simulink model "clock_recovery_3"  (Simulink 7.4)
settings: Solver=ode45  StartTime=0.0  StopTime=1e-5  MaxStep=.1/bit_rate  RelTol=1e-3
PreLoadFcn:
  | bit_rate=9.953e9;   % bits per second
libraries: simulink x7, dspsigops x6, dspsigattribs x4, commblksprivate x2, dspstat3 x2, commrandsrc2 x1, dspbuff3 x1, dspsnks4 x1
settings Model: Creator=dbenson  LastModifiedBy=Dick
settings SolverCC: ZeroCrossControl=EnableAll
settings OptimizationCC: InitFltsAndDblsToZero=on

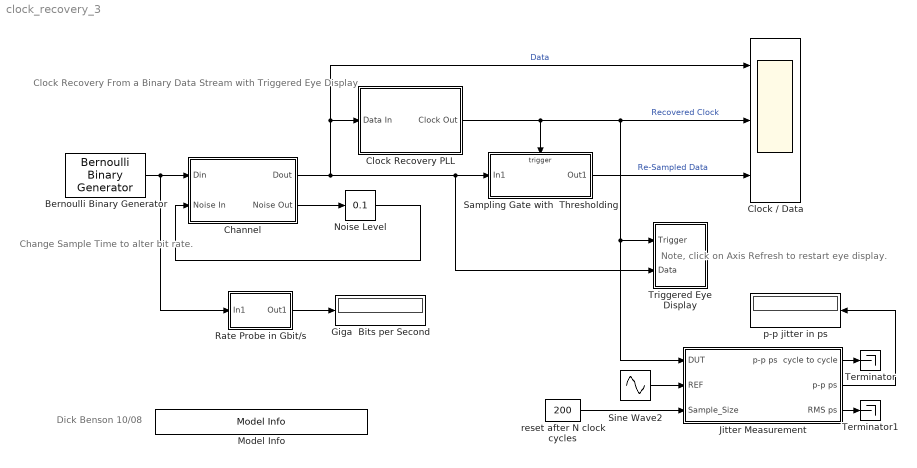
== system clock_recovery_3 ==
  note: Clock Recovery From a Binary Data Stream
      | with
      | Triggered Eye Display
  note: Note, click on Axis Refresh
      | to restart eye display.
  note: Dick Benson
      | 10/08
  note: Change Sample Time
      | to alter bit rate.
  Bernoulli Binary Generator : commrandsrc2/Bernoulli Binary Generator  DialogController=commDDGCreate  DialogControllerArgs=DataTag0  SystemSampleTime=-1  P=0.5  seed=21  Ts=1.001/ bit_rate  frameBased=off  sampPerFrame=1  orient=off  outDataType=boolean
  Channel : Subsystem
  "Clock / Data " : Scope  NumInputPorts=3
      settings: TimeRange=2.009444388626545e-010  YMin=-1~-0.2~-0.2  YMax=1~1.2~1.2
  Clock Recovery PLL : Subsystem
  Giga  Bits per Second : Display
  "Jitter Measurement " : Subsystem
  Model Info : simulink/Model-Wide Utilities/Model Info  SystemSampleTime=-1  InitialBlockCM=None  BlockCM=None  Frame=on  DisplayStringWithTags=Copywrite 2008-2010 The MathWorks, Inc.  HorizontalTextAlignment=Center  LeftAlignmentValue=0.5  SourceBlockDiagram=clock_recovery_3  TagMaxNumber=20
  Noise Level : simulink/Math Operations/Slider Gain  SystemSampleTime=-1  low=0  gain=0.1  high=1
  Rate Probe in Gbit/s : Subsystem
  Sampling Gate with  Thresholding : Subsystem
  Sine Wave2 : Sin  Amplitude=1  Bias=0  Frequency=2*pi*bit_rate  Phase=0  Samples=10  SampleTime=0  Offset=0
  Terminator : Terminator
  Terminator1 : Terminator
  Triggered Eye Display : Subsystem
  p-p jitter in ps : Display
  reset after N clock cycles : Constant  Value=200  VectorParams1D=off  OutDataType=sfix(16)  OutScaling=2^0
  wires:
  Clock Recovery PLL/1(Clock Out) -> Sampling Gate with  Thresholding/Trigger, "Clock / Data "/2, Triggered Eye Display/1(Trigger), "Jitter Measurement "/1(DUT)  "Recovered Clock"
  Bernoulli Binary Generator/1 -> Channel/1(Din), Rate Probe in Gbit/s/1(In1)
  Channel/1(Dout) -> Clock Recovery PLL/1(Data In), "Clock / Data "/1, Sampling Gate with  Thresholding/1(In1), Triggered Eye Display/2(Data)  "Data"
  Sampling Gate with  Thresholding/1(Out1) -> "Clock / Data "/3  "Re-Sampled Data"
  Rate Probe in Gbit/s/1(Out1) -> Giga  Bits per Second/1
  Sine Wave2/1 -> "Jitter Measurement "/2(REF)
  "Jitter Measurement "/2(p-p ps) -> p-p jitter in ps/1
  reset after N clock cycles/1 -> "Jitter Measurement "/3(Sample_Size)
  Channel/2(Noise Out) -> Noise Level/1
  Noise Level/1 -> Channel/2(Noise In)
  "Jitter Measurement "/1(p-p ps  cycle to cycle) -> Terminator/1
  "Jitter Measurement "/3(RMS ps) -> Terminator1/1

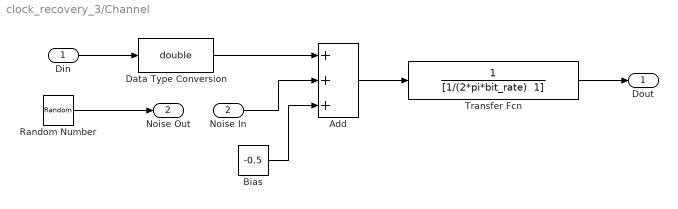
== system clock_recovery_3/Channel ==
  Din : Inport
  Noise In : Inport  Port=2
  Add : Sum  Inputs=+++  OutDataType=sfix(16)  OutScaling=2^-10
  Bias : Constant  Value=-0.5  OutDataType=sfix(16)  OutScaling=2^0
  Data Type Conversion : DataTypeConversion  OutDataTypeMode=double  OutDataType=sfix(16)  OutScaling=2^0  OutDataTypeStr=double
  Random Number : RandomNumber  SampleTime=0
  Transfer Fcn : TransferFcn  Denominator="[1/(2*pi*bit_rate)  1]"
  Dout : Outport
  Noise Out : Outport  Port=2
  wires:
  Din/1 -> Data Type Conversion/1
  Add/1 -> Transfer Fcn/1
  Data Type Conversion/1 -> Add/1
  Transfer Fcn/1 -> Dout/1
  Random Number/1 -> Noise Out/1
  Noise In/1 -> Add/2
  Bias/1 -> Add/3

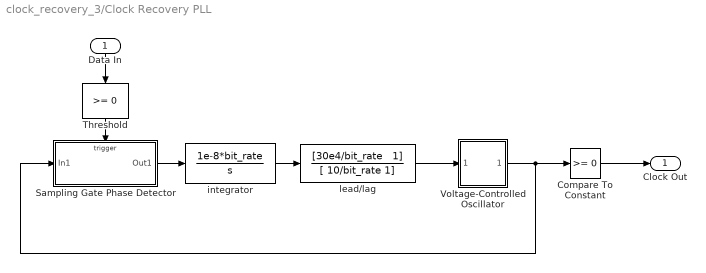
== system clock_recovery_3/Clock Recovery PLL ==
  Data In : Inport
  Compare To Constant : simulink/Logic and Bit Operations/Compare To Constant  SystemSampleTime=-1  relop=>=  const=0  LogicOutDataTypeMode=boolean  ZeroCross=off
  Sampling Gate Phase Detector : Subsystem
  Threshold : simulink/Logic and Bit Operations/Compare To Constant  SystemSampleTime=-1  relop=>=  const=0  LogicOutDataTypeMode=boolean  ZeroCross=off
  Voltage-Controlled Oscillator : Subsystem  mask(Voltage-Controlled Oscillator){Ac=1, Fc=bit_rate, Kc=bit_rate, Ph=0}
      mask prompts: Ac "Output amplitude:"; Fc "Oscillation frequency (Hz):"; Kc "Input sensitivity:"; Ph "Initial phase (rad):"
      mask help: Generate a continuous-time output signal whose frequency changes in response to the amplitude variations of the input signal. The input signal must be a sample-based scalar.
      mask init:
      | if ((length(Ac)~=1) | (length(Fc)~=1) | (length(Ph)~=1) | (length(Kc)~=1) )error('Mask parameters must be scalar values.');end;
      | pi2=2*pi;
      mask Help: helpview(commbhelp)
      mask Display: disp('VCO')
  integrator : TransferFcn  Numerator=1e-8*bit_rate  Denominator=[1 0]
  lead/lag : TransferFcn  Numerator="[30e4/bit_rate   1]"  Denominator=[ 10/bit_rate 1]
  Clock Out : Outport
  wires:
  lead/lag/1 -> Voltage-Controlled Oscillator/1(in_1)
  Voltage-Controlled Oscillator/1(out_1) -> Sampling Gate Phase Detector/1(In1), Compare To Constant/1
  integrator/1 -> lead/lag/1
  Sampling Gate Phase Detector/1(Out1) -> integrator/1
  Threshold/1 -> Sampling Gate Phase Detector/Trigger
  Data In/1 -> Threshold/1
  Compare To Constant/1 -> Clock Out/1

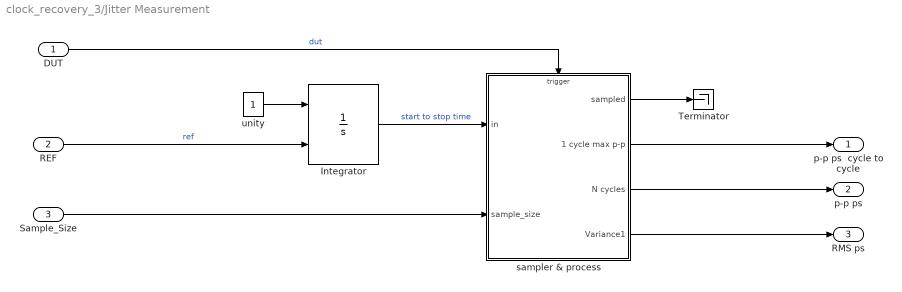
== system clock_recovery_3/Jitter Measurement  ==
  DUT : Inport  OutDataType=sfix(16)  OutScaling=2^0
  REF : Inport  Port=2  OutDataType=sfix(16)  OutScaling=2^0
  Sample_Size : Inport  Port=3  OutDataType=sfix(16)  OutScaling=2^0
  Integrator : Integrator  ExternalReset=rising
  Terminator : Terminator
  sampler & process : Subsystem  TreatAsAtomicUnit=on
  unity : Constant  OutDataTypeMode=double  OutDataType=sfix(16)  OutScaling=2^0  OutDataTypeStr=double
  p-p ps  cycle to cycle : Outport  OutDataType=sfix(16)  OutScaling=2^0
  p-p ps : Outport  Port=2  OutDataType=sfix(16)  OutScaling=2^0
  RMS ps : Outport  Port=3  OutDataType=sfix(16)  OutScaling=2^0
  wires:
  DUT/1 -> sampler & process/Trigger  "dut"
  REF/1 -> Integrator/2  "ref"
  Integrator/1 -> sampler & process/1(in)  "start to stop time"
  Sample_Size/1 -> sampler & process/2(sample_size)
  sampler & process/3(N cycles) -> p-p ps/1
  sampler & process/4(Variance1) -> RMS ps/1
  unity/1 -> Integrator/1
  sampler & process/2(1 cycle max p-p) -> p-p ps  cycle to cycle/1
  sampler & process/1(sampled) -> Terminator/1

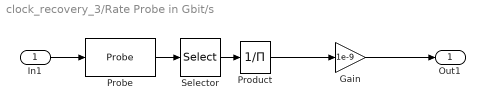
== system clock_recovery_3/Rate Probe in Gbit/s ==
  In1 : Inport
  Gain : Gain  Gain=1e-9  ParameterDataType=sfix(16)  ParameterScaling=2^0  OutDataType=sfix(16)  OutScaling=2^0
  Probe : Probe  ProbeWidth=off  ProbeComplexSignal=off
  Product : Product  Inputs=/  OutDataType=sfix(16)  OutScaling=2^0  RndMeth=Zero
  Selector : Selector  InputPortWidth=2  IndexOptions=Index vector (dialog)  Indices=[1]  OutputSizes=1
  Out1 : Outport
  wires:
  Probe/1 -> Selector/1
  Selector/1 -> Product/1
  In1/1 -> Probe/1
  Product/1 -> Gain/1
  Gain/1 -> Out1/1

== system clock_recovery_3/Sampling Gate with  Thresholding ==
  In1 : Inport  OutDataType=sfix(16)  OutScaling=2^0
  Trigger : TriggerPort
  Compare To Constant : simulink/Logic and Bit Operations/Compare To Constant  SystemSampleTime=-1  relop=>=  const=0  LogicOutDataTypeMode=boolean  ZeroCross=off
  Out1 : Outport  OutDataType=sfix(16)  OutScaling=2^0
  wires:
  In1/1 -> Compare To Constant/1
  Compare To Constant/1 -> Out1/1

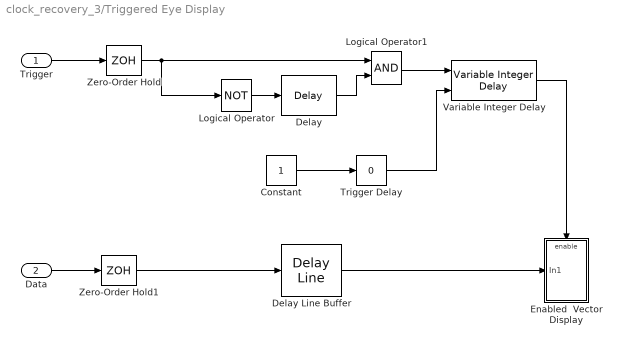
== system clock_recovery_3/Triggered Eye Display ==
  Trigger : Inport
  Data : Inport  Port=2
  Constant : Constant  OutDataType=sfix(16)  OutScaling=2^0
  Delay : dspsigops/Delay  dly_unit=Samples  delay=1  ic_detail=off  dif_ic_for_ch=off  dif_ic_for_dly=off  ic=0  reset_popup=None
  Delay Line Buffer : dspbuff3/Delay Line  siz=200  ic=0  directfeed=off  enable_output=off  hold_output=off
  Enabled  Vector Display : Subsystem
  Logical Operator : Logic  Operator=NOT  AllPortsSameDT=off  OutDataTypeMode=boolean  OutDataTypeStr=boolean
  Logical Operator1 : Logic  AllPortsSameDT=off  OutDataTypeMode=boolean  OutDataTypeStr=boolean
  Trigger Delay : simulink/Math Operations/Slider Gain  SystemSampleTime=-1  low=0  gain=0  high=100
  Variable Integer Delay : dspsigops/Variable Integer Delay  dmax=100  ic=0  noDFT=off
  Zero-Order Hold : ZeroOrderHold  SampleTime=.01/bit_rate
  Zero-Order Hold1 : ZeroOrderHold  SampleTime=.01/bit_rate
  wires:
  Zero-Order Hold/1 -> Logical Operator1/1, Logical Operator/1
  Logical Operator/1 -> Delay/1
  Delay/1 -> Logical Operator1/2
  Trigger/1 -> Zero-Order Hold/1
  Data/1 -> Zero-Order Hold1/1
  Zero-Order Hold1/1 -> Delay Line Buffer/1
  Delay Line Buffer/1 -> Enabled  Vector Display/1(In1)
  Logical Operator1/1 -> Variable Integer Delay/1
  Variable Integer Delay/1 -> Enabled  Vector Display/Enable
  Trigger Delay/1 -> Variable Integer Delay/2
  Constant/1 -> Trigger Delay/1

== system clock_recovery_3/Clock Recovery PLL/Sampling Gate Phase Detector ==
  In1 : Inport  OutDataType=sfix(16)  OutScaling=2^0
  Trigger : TriggerPort
  Out1 : Outport  OutDataType=sfix(16)  OutScaling=2^0
  wires:
  In1/1 -> Out1/1

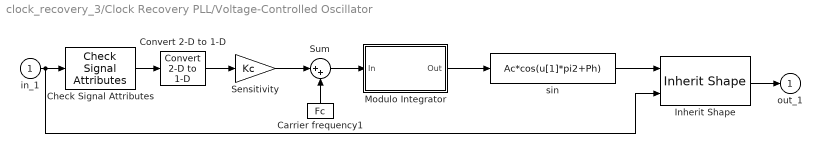
== system clock_recovery_3/Clock Recovery PLL/Voltage-Controlled Oscillator ==
  in_1 : Inport  OutDataType=sfix(16)  OutScaling=2^0
  Carrier frequency1 : Constant  Value=Fc  OutDataType=sfix(16)  OutScaling=2^0
  Check Signal Attributes : dspsigattribs/Check Signal Attributes  SystemSampleTime=-1  SigAttribCheckMethod=Does not match attributes exactly  Complexity=Ignore  Frame=Sample-based  DimsCheckMethod=Is...  Dimensions=Scalar (1-D or 2-D)  DatatypeCheckMethod=Ignore  DatatypeGeneral=Boolean  DtypeFloatSpecific=Any floating-point  DtypeFixedSpecific=Any fixed-point  DtypeIntSpecific=Any integer  SampleMode=Ignore
  Convert 2-D to 1-D : dspsigattribs/Convert 2-D to 1-D  SystemSampleTime=-1
  Inherit Shape : commblksprivate/Inherit Shape
  Modulo Integrator : Subsystem  mask(Modulo Integrator){modu=1, init=0}
      mask prompts: modu "Absolute value bound:"; init "Initial condition:"
      mask help:
      | Integrate the input signal in continuous time and then uses the Absolute value bound parameter, K, to produce output strictly between -K and K. The block uses the rem function in MATLAB.
      |
      | The input must be sample-based.
      mask init:
      | [modu, init]=commblkmodint(gcb);
      mask Help: helpview(commbhelp)
      mask Display: disp('Modulo\nIntegrator')
  Sensitivity : Gain  Gain=Kc  ParameterDataType=sfix(16)  ParameterScaling=2^0  OutDataType=sfix(16)  OutScaling=2^0  SaturateOnIntegerOverflow=on  OutDataTypeStr=Inherit: Same as input  ParamDataTypeStr=Inherit: Same as input
  Sum : Sum  Inputs=|++  OutDataType=sfix(16)  OutScaling=2^0  SaturateOnIntegerOverflow=on  InputSameDT=on  OutDataTypeStr=Inherit: Same as first input
  sin : Fcn  Expr=Ac*cos(u[1]*pi2+Ph)
  out_1 : Outport  OutDataType=sfix(16)  OutScaling=2^0  InitialOutput=0
  wires:
  Check Signal Attributes/1 -> Convert 2-D to 1-D/1
  Inherit Shape/1 -> out_1/1
  sin/1 -> Inherit Shape/1
  Convert 2-D to 1-D/1 -> Sensitivity/1
  in_1/1 -> Check Signal Attributes/1, Inherit Shape/2
  Sensitivity/1 -> Sum/1
  Carrier frequency1/1 -> Sum/2
  Modulo Integrator/1(Out) -> sin/1
  Sum/1 -> Modulo Integrator/1(In)

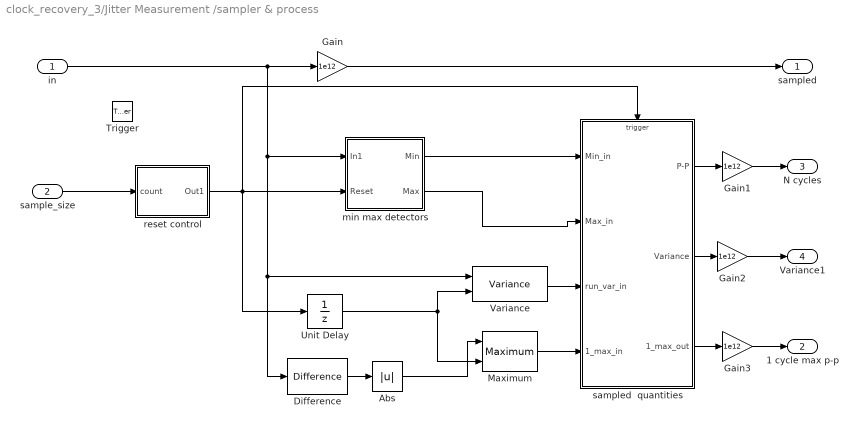
== system clock_recovery_3/Jitter Measurement /sampler & process ==
  in : Inport  OutDataType=sfix(16)  OutScaling=2^0
  sample_size : Inport  Port=2  OutDataType=sfix(16)  OutScaling=2^0
  Trigger : TriggerPort
  Abs : Abs
  Difference : simulink/Discrete/Difference  SystemSampleTime=-1  ICPrevInput=0.0  OutMin=[]  OutMax=[]  OutDataType=sfix(16)  OutScaling=2^-10  DoSatur=off
  Gain{,1..3} (4 alike) : Gain  Gain=1e12  ParameterDataType=sfix(16)  ParameterScaling=2^0  OutDataType=sfix(16)  OutScaling=2^0
  Maximum : dspstat3/Maximum  DialogController=dspDDGCreate  DialogControllerArgs=DataTag1  fcn=Running  reset=Rising edge  indexBase=One  operateOver=Each column  Dimension=1  colComp=on  operation=maximum  roiEnable=off  roiType=Rectangles  roiPortion=Entire ROI  roiOutput=Individual statistics for each ROI  roiFlag=off  accumDataTypeStr=Inherit: Same as product output  accumLastDataTypeStr=Inherit: Same as product output  roundingMode=Floor  overflowMode=off
  Unit Delay : UnitDelay  SampleTime=-1
  Variance : dspstat3/Variance  DialogController=dspDDGCreate  DialogControllerArgs=DataTag2  run=on  reset_popup=Rising edge  directionMode=Each column  dimension=1  treatSBRowAsCol=on  roiEnable=off  roiType=Rectangles  roiPortion=Entire ROI  roiOutput=Individual statistics for each ROI  roiFlag=off  roundingMode=Floor  overflowMode=off
  min max detectors : Subsystem
  reset control : Subsystem
  sampled  quantities : Subsystem  TreatAsAtomicUnit=on
  sampled : Outport  OutDataType=sfix(16)  OutScaling=2^0
  1 cycle max p-p : Outport  Port=2  OutDataType=sfix(16)  OutScaling=2^0
  N cycles : Outport  Port=3  OutDataType=sfix(16)  OutScaling=2^0
  Variance1 : Outport  Port=4  OutDataType=sfix(16)  OutScaling=2^0
  wires:
  in/1 -> Gain/1, Variance/1, Difference/1, min max detectors/1(In1)
  Difference/1 -> Abs/1
  Abs/1 -> Maximum/1
  sample_size/1 -> reset control/1(count)
  reset control/1(Out1) -> Unit Delay/1, sampled  quantities/Trigger, min max detectors/2(Reset)
  sampled  quantities/1(P-P) -> Gain1/1
  Variance/1 -> sampled  quantities/3(run_var_in)
  sampled  quantities/2(Variance) -> Gain2/1
  Unit Delay/1 -> Variance/2, Maximum/2
  Maximum/1 -> sampled  quantities/4(1_max_in)
  sampled  quantities/3(1_max_out) -> Gain3/1
  Gain/1 -> sampled/1
  Gain1/1 -> N cycles/1
  Gain2/1 -> Variance1/1
  Gain3/1 -> 1 cycle max p-p/1
  min max detectors/2(Max) -> sampled  quantities/2(Max_in)
  min max detectors/1(Min) -> sampled  quantities/1(Min_in)

== system clock_recovery_3/Triggered Eye Display/Enabled  Vector Display ==
  In1 : Inport
  Enable : EnablePort
  Vector Scope1 : dspsnks4/Vector Scope  DialogController=dspdialog.VectorScope  DialogControllerArgs=DataTag3  ScopeProperties=on  Domain=User-defined  HorizSpan=1  DisplayProperties=off  AxisGrid=on  Memory=on  FrameNumber=on  AxisLegend=off  AxisZoom=off  OpenScopeAtSimStart=on  OpenScopeImmediately=off  FigPos=[9 30 411 270]  AxisProperties=off  XUnits=Hertz  XRange=[0...Fs/2]  InheritXIncr=off  XIncr=.01/bit_rate  XLabel=Time  XLimit=Auto  XMin=0  XMax=1  XStart=0  YUnits=dB  YLabel=Amplitude  LineProperties=off  LineColors=[0 0 1]|[1 0 0]  XAxisParamsVer=6.8
      settings: YMin=-.7  YMax=.7
  wires:
  In1/1 -> Vector Scope1/1

== system clock_recovery_3/Clock Recovery PLL/Voltage-Controlled Oscillator/Modulo Integrator ==
  In : Inport  OutDataType=sfix(16)  OutScaling=2^0
  "Exclude Frame-based Input " : dspsigattribs/Check Signal Attributes  SystemSampleTime=-1  SigAttribCheckMethod=Matches attributes exactly  Complexity=Ignore  Frame=Frame-based  DimsCheckMethod=Ignore  Dimensions=Scalar (1-D or 2-D)  DatatypeCheckMethod=Ignore  DatatypeGeneral=Boolean  DtypeFloatSpecific=Any floating-point  DtypeFixedSpecific=Any fixed-point  DtypeIntSpecific=Any integer  SampleMode=Ignore
  Exclude Full Matrix : dspsigattribs/Check Signal Attributes  SystemSampleTime=-1  SigAttribCheckMethod=Matches attributes exactly  Complexity=Ignore  Frame=Ignore  DimsCheckMethod=Is...  Dimensions=Full matrix (2-D)  DatatypeCheckMethod=Ignore  DatatypeGeneral=Boolean  DtypeFloatSpecific=Any floating-point  DtypeFixedSpecific=Any fixed-point  DtypeIntSpecific=Any integer  SampleMode=Ignore
  Inherit Shape : commblksprivate/Inherit Shape
  Modulo Integrator : Subsystem
  Out : Outport  OutDataType=sfix(16)  OutScaling=2^0
  wires:
  Exclude Full Matrix/1 -> "Exclude Frame-based Input "/1
  "Exclude Frame-based Input "/1 -> Modulo Integrator/1(In1)
  In/1 -> Exclude Full Matrix/1, Inherit Shape/2
  Modulo Integrator/1(Out1) -> Inherit Shape/1
  Inherit Shape/1 -> Out/1

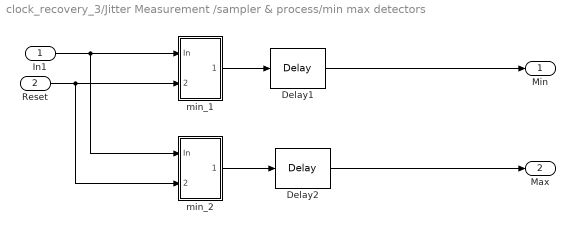
== system clock_recovery_3/Jitter Measurement /sampler & process/min max detectors ==
  In1 : Inport  OutDataType=sfix(16)  OutScaling=2^0
  Reset : Inport  Port=2  OutDataType=sfix(16)  OutScaling=2^0
  Delay1 : dspsigops/Delay  dly_unit=Samples  delay=1  ic_detail=off  dif_ic_for_ch=off  dif_ic_for_dly=off  ic=0  reset_popup=None
  Delay2 : dspsigops/Delay  dly_unit=Samples  delay=1  ic_detail=off  dif_ic_for_ch=off  dif_ic_for_dly=off  ic=0  reset_popup=None
  min_1 : Subsystem
  min_2 : Subsystem
  Min : Outport  OutDataType=sfix(16)  OutScaling=2^0
  Max : Outport  Port=2  OutDataType=sfix(16)  OutScaling=2^0
  wires:
  Reset/1 -> min_1/2(Rst), min_2/2(Rst)
  In1/1 -> min_1/1(In), min_2/1(In)
  min_1/1(Out) -> Delay1/1
  min_2/1(Out) -> Delay2/1
  Delay1/1 -> Min/1
  Delay2/1 -> Max/1

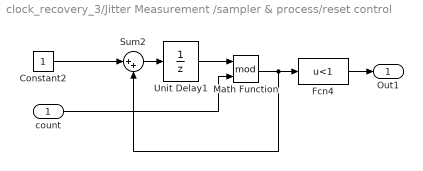
== system clock_recovery_3/Jitter Measurement /sampler & process/reset control ==
  count : Inport  OutDataType=sfix(16)  OutScaling=2^0
  Constant2 : Constant  OutDataType=sfix(16)  OutScaling=2^0
  Fcn4 : Fcn  Expr=u<1
  Math Function : Math  Operator=mod  OutDataType=sfix(16)  OutScaling=2^0  SaturateOnIntegerOverflow=on
  Sum2 : Sum  Inputs=|++  OutDataType=sfix(16)  OutScaling=2^0  SaturateOnIntegerOverflow=on  InputSameDT=on  OutDataTypeStr=Inherit: Same as first input
  Unit Delay1 : UnitDelay  SampleTime=-1
  Out1 : Outport  OutDataType=sfix(16)  OutScaling=2^0
  wires:
  Math Function/1 -> Fcn4/1, Sum2/2
  Unit Delay1/1 -> Math Function/1
  Constant2/1 -> Sum2/1
  Sum2/1 -> Unit Delay1/1
  Fcn4/1 -> Out1/1
  count/1 -> Math Function/2

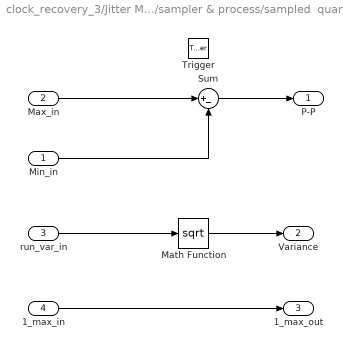
== system clock_recovery_3/Jitter Measurement /sampler & process/sampled  quantities ==
  Min_in : Inport  OutDataType=sfix(16)  OutScaling=2^0
  Max_in : Inport  Port=2  OutDataType=sfix(16)  OutScaling=2^0
  run_var_in : Inport  Port=3  OutDataType=sfix(16)  OutScaling=2^0
  1_max_in : Inport  Port=4  OutDataType=sfix(16)  OutScaling=2^0
  Trigger : TriggerPort
  Math Function : Math  Operator=sqrt  OutDataType=sfix(16)  OutScaling=2^0  SaturateOnIntegerOverflow=on
  Sum : Sum  Inputs=|+-  OutDataType=sfix(16)  OutScaling=2^0  SaturateOnIntegerOverflow=on  InputSameDT=on  OutDataTypeStr=Inherit: Same as first input
  P-P : Outport  OutDataType=sfix(16)  OutScaling=2^0
  Variance : Outport  Port=2  OutDataType=sfix(16)  OutScaling=2^0
  1_max_out : Outport  Port=3  OutDataType=sfix(16)  OutScaling=2^0
  wires:
  Max_in/1 -> Sum/1
  Min_in/1 -> Sum/2
  Sum/1 -> P-P/1
  Math Function/1 -> Variance/1
  run_var_in/1 -> Math Function/1
  1_max_in/1 -> 1_max_out/1

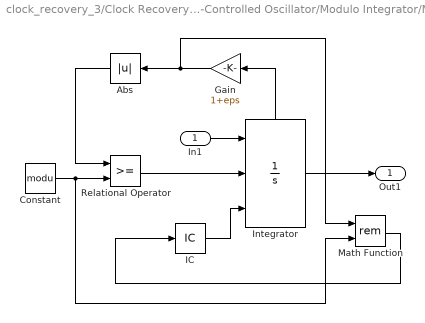
== system clock_recovery_3/Clock Recovery PLL/Voltage-Controlled Oscillator/Modulo Integrator/Modulo Integrator ==
  In1 : Inport  OutDataType=sfix(16)  OutScaling=2^0
  Abs : Abs  OutDataType=sfix(16)  OutScaling=2^0  SaturateOnIntegerOverflow=on
  Constant : Constant  Value=modu  OutDataType=sfix(16)  OutScaling=2^0
  Gain : Gain  Gain=1+eps  ParameterDataType=sfix(16)  ParameterScaling=2^0  OutDataType=sfix(16)  OutScaling=2^0  SaturateOnIntegerOverflow=on  OutDataTypeStr=Inherit: Same as input  ParamDataTypeStr=Inherit: Same as input
  IC : InitialCondition  Value=init
  Integrator : Integrator  ExternalReset=rising  InitialConditionSource=external  UpperSaturationLimit=1  LowerSaturationLimit=0  ShowStatePort=on
  Math Function : Math  Operator=rem  OutDataType=sfix(16)  OutScaling=2^0  SaturateOnIntegerOverflow=on
  Relational Operator : RelationalOperator  InputSameDT=on
  Out1 : Outport  OutDataType=sfix(16)  OutScaling=2^0
  wires:
  IC/1 -> Integrator/3
  In1/1 -> Integrator/1
  Integrator/1 -> Out1/1
  Math Function/1 -> IC/1
  Abs/1 -> Relational Operator/1
  Relational Operator/1 -> Integrator/2
  Constant/1 -> Math Function/2, Relational Operator/2
  Integrator/State -> Gain/1
  Gain/1 -> Abs/1, Math Function/1

== system clock_recovery_3/Jitter Measurement /sampler & process/min max detectors/min_1 ==
  In : Inport  OutDataType=sfix(16)  OutScaling=2^0
  Rst : Inport  Port=2  OutDataType=sfix(16)  OutScaling=2^0
  Delay : dspsigops/Delay  dly_unit=Samples  delay=1  ic_detail=off  dif_ic_for_ch=off  dif_ic_for_dly=off  ic=1e6  reset_popup=Non-zero sample
  Relational Operator : RelationalOperator  Operator=<  LogicOutDataTypeMode=boolean  OutDataTypeStr=boolean
  Switch : Switch  Threshold=.5
  Out : Outport  OutDataType=sfix(16)  OutScaling=2^0
  wires:
  In/1 -> Relational Operator/1, Switch/1
  Rst/1 -> Delay/2
  Delay/1 -> Relational Operator/2, Switch/3
  Relational Operator/1 -> Switch/2
  Switch/1 -> Delay/1, Out/1

== system clock_recovery_3/Jitter Measurement /sampler & process/min max detectors/min_2 ==
  In : Inport  OutDataType=sfix(16)  OutScaling=2^0
  Rst : Inport  Port=2  OutDataType=sfix(16)  OutScaling=2^0
  Delay : dspsigops/Delay  dly_unit=Samples  delay=1  ic_detail=off  dif_ic_for_ch=off  dif_ic_for_dly=off  ic=-1e6  reset_popup=Non-zero sample
  Relational Operator : RelationalOperator  Operator=>  LogicOutDataTypeMode=boolean  OutDataTypeStr=boolean
  Switch : Switch  Threshold=.5
  Out : Outport  OutDataType=sfix(16)  OutScaling=2^0
  wires:
  Switch/1 -> Out/1, Delay/1
  Relational Operator/1 -> Switch/2
  Delay/1 -> Switch/3, Relational Operator/2
  Rst/1 -> Delay/2
  In/1 -> Switch/1, Relational Operator/1
